simulink model "slrt_induction_2level_inverter"  (R2022b)
settings: Solver=FixedStepAuto  StartTime=0.0  StopTime=0.25  RelTol=1e-3  EnableMultiTasking=on
PreLoadFcn:
  | Ts = 1e-4;
  | Tcpu = 50e-6; %Controller sample time
  | 
  | % PMSM parameters
  | PM = 0.03; % Permanent magnet flux linkage
  | Ld = 2e-4;  % d-axis inductance
  | Lq = 2e-4;  % q-axis inductance
  | L0 = 2e-4;  % 0-axis inductance
  | Rs = 0.013; % Stator resistance
  | N = 6; % Number of pole pairs
  | J = 0.2; % Moment of inertia
  | 
  | % encoder parameters
  | numSlits = 2000; % number of slits
  | pulseSigOffset = 0; % index pulse signal offset
  | shaftInitPos = 0; % motor shaft initial position
  | 
  | % DAC parameters
  | gain = 0.1;
  | bias = 0;
  | 
  | % circuit parameters
  | Vdc = 48;
  | 
  | % real-time parameters
  | ts_FPGA_clk = 5e-9;
  | ts_FPGA_mdl = 1e-6;
  | 
  | % Real-time processor or embedded controller
  | RTorTTL = 1; % 1: Real-time processor,    0: embedded controller
  | 
  | % sample times
  | f_base = 200e6;
  | PWM_frequency = 20e3;
  | ts_FPGA_clk = 1/f_base;
  | ts_FPGA_mdl =1e-6;
undefined symbols (not defined in the file or in its folder): DiscIntNeverNeededParam
libraries: simulink x7, hdlsllib x3, slrtencoderlib x2, slrtresolverlib x2, mcbhdlplantlib x1, slrthdlutillib x1, slrt2levelinverterlib x1
(part 1 of 2)
settings Model: Creator=chrisz  LastModifiedBy=chrisz
settings OptimizationCC: BlockReduction=off  ConditionallyExecuteInputs=off  DefaultParameterBehavior=Inlined
settings DebuggingCC: AlgebraicLoopMsg=error  SingleTaskRateTransMsg=error
settings HardwareCC: ProdBitPerPointer=32  ProdBitPerSizeT=32  ProdBitPerPtrDiffT=32  ProdLargestAtomicFloat=None  ProdIntDivRoundTo=Undefined  ProdEndianess=Unspecified  ProdWordSize=32  ProdHWDeviceType=ASIC/FPGA->ASIC/FPGA  TargetBitPerPointer=64  TargetBitPerSizeT=64  TargetBitPerPtrDiffT=64  TargetLongLongMode=on  TargetIntDivRoundTo=Zero  TargetEndianess=LittleEndian  TargetWordSize=64  TargetHWDeviceType=Custom Processor->MATLAB Host Computer  ProdEqTarget=off
settings ModelReferenceCC: EnableRefExpFcnMdlSchedulingChecks=on

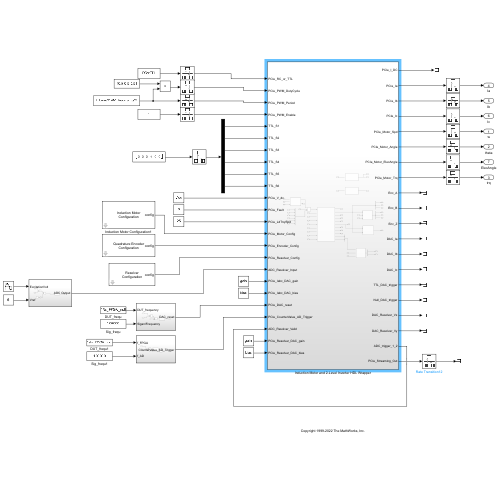
[thumbnail: Simulink's stored preview of the top-level diagram]
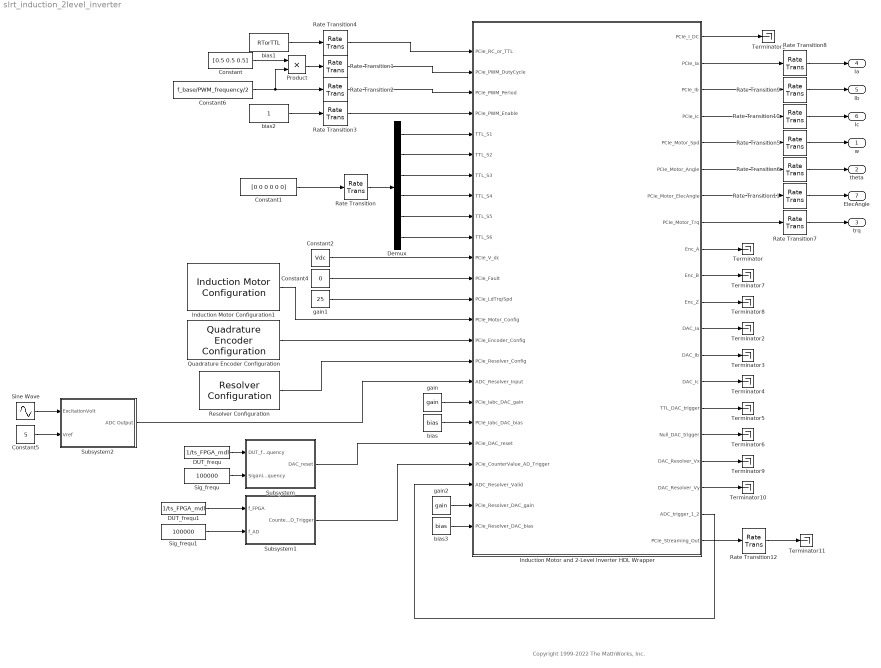
== system slrt_induction_2level_inverter ==
  note: Copyright 1999-2022 The MathWorks, Inc.
  Constant : Constant  Value=[0.5 0.5 0.5]  OutDataTypeStr=single  SampleTime=ts_FPGA_mdl
  Constant1 : Constant  Value=[0 0 0 0 0 0]  OutDataTypeStr=boolean  SampleTime=-1
  Constant2 : Constant  Value=Vdc  OutDataTypeStr=single  SampleTime=ts_FPGA_mdl
  Constant4 : Constant  Value=0  OutDataTypeStr=uint32  SampleTime=ts_FPGA_mdl
  Constant5 : Constant  Value=5  SampleTime=ts_FPGA_mdl
  Constant6 : Constant  Value=f_base/PWM_frequency/2  OutDataTypeStr=uint32  SampleTime=ts_FPGA_mdl
  DUT_frequ : Constant  Value=1/ts_FPGA_mdl  SampleTime=ts_FPGA_mdl
  DUT_frequ1 : Constant  Value=1/ts_FPGA_mdl  SampleTime=ts_FPGA_mdl
  Demux : Demux  Outputs=6
  Induction Motor Configuration1 : mcbhdlplantlib/Induction Motor Configuration  portConfig=Torque  Tw_mode=0  Ts=1e-6  P=2  Rs=1.77  Lls=0.0139  Rr=1.34  Llr=0.0121  Lm=0.3876  J=0.001  B=0  f=0
  Induction Motor and 2-Level Inverter HDL Wrapper : Subsystem
  Product : Product  OutDataTypeStr=uint32
  Quadrature Encoder Configuration : slrtencoderlib/Quadrature Encoder Configuration  NPulses=2000  zOffset=0  Ts=1e-6
  Rate Transition{,1..4} (5 alike) : RateTransition  OutPortSampleTime=ts_FPGA_clk
  Rate Transition{5..12} (8 alike) : RateTransition  OutPortSampleTime=Tcpu
  Resolver Configuration : slrtresolverlib/Resolver Configuration  Ts=1e-6  R=0.5  N=1  ADCrefV=5  ADCbits=12  totalADCCounts=4096
  Sig_frequ : Constant  Value=100000  VectorParams1D=off  SampleTime=ts_FPGA_mdl
  Sig_frequ1 : Constant  Value=100000  VectorParams1D=off  SampleTime=ts_FPGA_mdl
  Sine Wave : Sin  Amplitude=5  Frequency=62830  SampleTime=ts_FPGA_mdl
  Subsystem : Subsystem
  Subsystem1 : Subsystem
  Subsystem2 : Subsystem
  Terminator{,1..11} (12 alike) : Terminator
  bias : Constant  Value=bias  OutDataTypeStr=single  SampleTime=ts_FPGA_mdl
  bias1 : Constant  Value=RTorTTL  OutDataTypeStr=single  SampleTime=ts_FPGA_mdl
  bias2 : Constant  OutDataTypeStr=boolean  SampleTime=ts_FPGA_mdl
  bias3 : Constant  Value=bias  OutDataTypeStr=single  SampleTime=ts_FPGA_mdl
  gain : Constant  Value=gain  OutDataTypeStr=single  SampleTime=ts_FPGA_mdl
  gain1 : Constant  Value=25  OutDataTypeStr=single  SampleTime=ts_FPGA_mdl
  gain2 : Constant  Value=gain  OutDataTypeStr=single  SampleTime=ts_FPGA_mdl
  w : Outport
  theta : Outport  Port=2
  trq : Outport  Port=3
  Ia : Outport  Port=4
  Ib : Outport  Port=5
  Ic : Outport  Port=6
  ElecAngle : Outport  Port=7
  wires:
  bias1/1 -> Rate Transition4/1
  bias2/1 -> Rate Transition3/1
  Constant6/1 -> Product/2, Rate Transition2/1
  Product/1 -> Rate Transition1/1
  Constant/1 -> Product/1
  gain/1 -> Induction Motor and 2-Level Inverter HDL Wrapper/18(PCIe_Iabc_DAC_gain)
  bias/1 -> Induction Motor and 2-Level Inverter HDL Wrapper/19(PCIe_Iabc_DAC_bias)
  Rate Transition4/1 -> Induction Motor and 2-Level Inverter HDL Wrapper/1(PCIe_RC_or_TTL)
  Rate Transition3/1 -> Induction Motor and 2-Level Inverter HDL Wrapper/4(PCIe_PWM_Enable)
  Rate Transition2/1 -> Induction Motor and 2-Level Inverter HDL Wrapper/3(PCIe_PWM_Period)
  Rate Transition1/1 -> Induction Motor and 2-Level Inverter HDL Wrapper/2(PCIe_PWM_DutyCycle)
  Rate Transition/1 -> Demux/1
  Demux/1 -> Induction Motor and 2-Level Inverter HDL Wrapper/5(TTL_S1)
  Demux/2 -> Induction Motor and 2-Level Inverter HDL Wrapper/6(TTL_S2)
  Demux/3 -> Induction Motor and 2-Level Inverter HDL Wrapper/7(TTL_S3)
  Demux/4 -> Induction Motor and 2-Level Inverter HDL Wrapper/8(TTL_S4)
  Demux/5 -> Induction Motor and 2-Level Inverter HDL Wrapper/9(TTL_S5)
  Demux/6 -> Induction Motor and 2-Level Inverter HDL Wrapper/10(TTL_S6)
  Constant1/1 -> Rate Transition/1
  Constant2/1 -> Induction Motor and 2-Level Inverter HDL Wrapper/11(PCIe_V_dc)
  Constant4/1 -> Induction Motor and 2-Level Inverter HDL Wrapper/12(PCIe_Fault)
  gain1/1 -> Induction Motor and 2-Level Inverter HDL Wrapper/13(PCIe_LdTrq/Spd)
  DUT_frequ/1 -> Subsystem/1(DUT_frequency)
  Sig_frequ/1 -> Subsystem/2(SiganlFrequency)
  Subsystem/1(DAC_reset) -> Induction Motor and 2-Level Inverter HDL Wrapper/20(PCIe_DAC_reset)
  Rate Transition6/1 -> theta/1
  Induction Motor and 2-Level Inverter HDL Wrapper/9(Enc_A) -> Terminator/1
  Rate Transition7/1 -> trq/1
  Induction Motor and 2-Level Inverter HDL Wrapper/12(DAC_Ia) -> Terminator2/1
  Induction Motor and 2-Level Inverter HDL Wrapper/1(PCIe_I_DC) -> Terminator1/1
  Induction Motor and 2-Level Inverter HDL Wrapper/10(Enc_B) -> Terminator7/1
  Induction Motor and 2-Level Inverter HDL Wrapper/14(DAC_Ic) -> Terminator4/1
  Rate Transition5/1 -> w/1
  Rate Transition10/1 -> Ic/1
  Induction Motor and 2-Level Inverter HDL Wrapper/15(TTL_DAC_trigger) -> Terminator5/1
  Induction Motor and 2-Level Inverter HDL Wrapper/13(DAC_Ib) -> Terminator3/1
  Induction Motor and 2-Level Inverter HDL Wrapper/16(Null_DAC_trigger) -> Terminator6/1
  Rate Transition9/1 -> Ib/1
  Rate Transition8/1 -> Ia/1
  Induction Motor and 2-Level Inverter HDL Wrapper/5(PCIe_Motor_Spd) -> Rate Transition5/1
  Induction Motor and 2-Level Inverter HDL Wrapper/6(PCIe_Motor_Angle) -> Rate Transition6/1
  Induction Motor and 2-Level Inverter HDL Wrapper/8(PCIe_Motor_Trq) -> Rate Transition7/1
  Induction Motor and 2-Level Inverter HDL Wrapper/2(PCIe_Ia) -> Rate Transition8/1
  Induction Motor and 2-Level Inverter HDL Wrapper/3(PCIe_Ib) -> Rate Transition9/1
  Induction Motor and 2-Level Inverter HDL Wrapper/4(PCIe_Ic) -> Rate Transition10/1
  Induction Motor and 2-Level Inverter HDL Wrapper/11(Enc_Z) -> Terminator8/1
  Induction Motor and 2-Level Inverter HDL Wrapper/17(DAC_Resolver_Vx) -> Terminator9/1
  Induction Motor and 2-Level Inverter HDL Wrapper/18(DAC_Resolver_Vy) -> Terminator10/1
  Quadrature Encoder Configuration/1 -> Induction Motor and 2-Level Inverter HDL Wrapper/15(PCIe_Encoder_Config)
  Induction Motor Configuration1/1 -> Induction Motor and 2-Level Inverter HDL Wrapper/14(PCIe_Motor_Config)
  Resolver Configuration/1 -> Induction Motor and 2-Level Inverter HDL Wrapper/16(PCIe_Resolver_Config)
  Subsystem1/1(CounterValue_AD_Trigger) -> Induction Motor and 2-Level Inverter HDL Wrapper/21(PCIe_CounterValue_AD_Trigger)
  Induction Motor and 2-Level Inverter HDL Wrapper/19(ADC_trigger_1_2) -> Induction Motor and 2-Level Inverter HDL Wrapper/22(ADC_Resolver_Valid)
  Sig_frequ1/1 -> Subsystem1/2(f_AD)
  DUT_frequ1/1 -> Subsystem1/1(f_FPGA)
  Sine Wave/1 -> Subsystem2/1(ExcitationVolt)
  Constant5/1 -> Subsystem2/2(Vref)
  Subsystem2/1(ADC Output) -> Induction Motor and 2-Level Inverter HDL Wrapper/17(ADC_Resolver_Input)
  Rate Transition11/1 -> ElecAngle/1
  Induction Motor and 2-Level Inverter HDL Wrapper/7(PCIe_Motor_ElecAngle) -> Rate Transition11/1
  gain2/1 -> Induction Motor and 2-Level Inverter HDL Wrapper/23(PCIe_Resolver_DAC_gain)
  bias3/1 -> Induction Motor and 2-Level Inverter HDL Wrapper/24(PCIe_Resolver_DAC_bias)
  Induction Motor and 2-Level Inverter HDL Wrapper/20(PCIe_Streaming_Out) -> Rate Transition12/1
  Rate Transition12/1 -> Terminator11/1

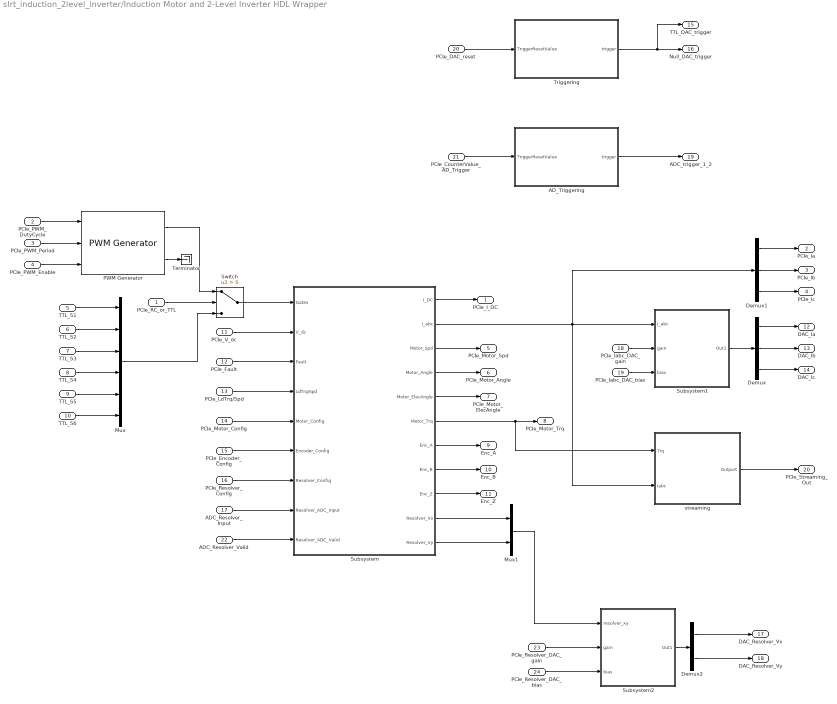
== system slrt_induction_2level_inverter/Induction Motor and 2-Level Inverter HDL Wrapper ==
  PCIe_RC_or_TTL : Inport
  PCIe_PWM_DutyCycle : Inport  Port=2
  PCIe_PWM_Period : Inport  Port=3
  PCIe_PWM_Enable : Inport  Port=4
  TTL_S1 : Inport  Port=5
  TTL_S2 : Inport  Port=6
  TTL_S3 : Inport  Port=7
  TTL_S4 : Inport  Port=8
  TTL_S5 : Inport  Port=9
  TTL_S6 : Inport  Port=10
  PCIe_V_dc : Inport  Port=11
  PCIe_Fault : Inport  Port=12
  PCIe_LdTrq/Spd : Inport  Port=13
  PCIe_Motor_Config : Inport  Port=14
  PCIe_Encoder_Config : Inport  Port=15
  PCIe_Resolver_Config : Inport  Port=16
  ADC_Resolver_Input : Inport  Port=17
  PCIe_Iabc_DAC_gain : Inport  Port=18
  PCIe_Iabc_DAC_bias : Inport  Port=19
  PCIe_DAC_reset : Inport  Port=20
  PCIe_CounterValue_AD_Trigger : Inport  Port=21  OutDataTypeStr=uint32
  ADC_Resolver_Valid : Inport  Port=22
  PCIe_Resolver_DAC_gain : Inport  Port=23
  PCIe_Resolver_DAC_bias : Inport  Port=24
  AD_Triggering : Subsystem
  Demux : Demux  Outputs=3
  Demux1 : Demux  Outputs=3
  Demux2 : Demux  Outputs=2
  Mux : Mux  Inputs=6
  Mux1 : Mux  Inputs=2
  PWM Generator : slrthdlutillib/PWM Generator
  Subsystem : Subsystem
  Subsystem1 : Subsystem
  Subsystem2 : Subsystem
  Switch : Switch  Criteria=u2 > Threshold  SaturateOnIntegerOverflow=off  InputSameDT=off
  Terminator : Terminator
  Triggering : Subsystem
  streaming : Subsystem
  PCIe_I_DC : Outport
  PCIe_Ia : Outport  Port=2
  PCIe_Ib : Outport  Port=3
  PCIe_Ic : Outport  Port=4
  PCIe_Motor_Spd : Outport  Port=5
  PCIe_Motor_Angle : Outport  Port=6
  PCIe_Motor_ElecAngle : Outport  Port=7
  PCIe_Motor_Trq : Outport  Port=8
  Enc_A : Outport  Port=9
  Enc_B : Outport  Port=10
  Enc_Z : Outport  Port=11
  DAC_Ia : Outport  Port=12
  DAC_Ib : Outport  Port=13
  DAC_Ic : Outport  Port=14
  TTL_DAC_trigger : Outport  Port=15
  Null_DAC_trigger : Outport  Port=16
  DAC_Resolver_Vx : Outport  Port=17
  DAC_Resolver_Vy : Outport  Port=18
  ADC_trigger_1_2 : Outport  Port=19  OutDataTypeStr=boolean
  PCIe_Streaming_Out : Outport  Port=20
  wires:
  Subsystem/7(Enc_A) -> Enc_A/1
  TTL_S2/1 -> Mux/2
  Demux1/1 -> PCIe_Ia/1
  PCIe_PWM_DutyCycle/1 -> PWM Generator/1
  TTL_S5/1 -> Mux/5
  Subsystem/2(I_abc) -> Demux1/1, streaming/2(Iabc), Subsystem1/1(I_abc)
  Subsystem/6(Motor_Trq) -> streaming/1(Trq), PCIe_Motor_Trq/1
  Subsystem/4(Motor_Angle) -> PCIe_Motor_Angle/1
  Subsystem/1(I_DC) -> PCIe_I_DC/1
  PCIe_Encoder_Config/1 -> Subsystem/6(Encoder_Config)
  PCIe_Iabc_DAC_bias/1 -> Subsystem1/3(bias)
  Subsystem/3(Motor_Spd) -> PCIe_Motor_Spd/1
  Subsystem/8(Enc_B) -> Enc_B/1
  PCIe_V_dc/1 -> Subsystem/2(V_dc)
  PWM Generator/1 -> Switch/1
  Triggering/1(trigger) -> Null_DAC_trigger/1, TTL_DAC_trigger/1
  TTL_S6/1 -> Mux/6
  Subsystem/9(Enc_Z) -> Enc_Z/1
  PCIe_LdTrq/Spd/1 -> Subsystem/4(LdTrq/Spd)
  TTL_S1/1 -> Mux/1
  Demux1/3 -> PCIe_Ic/1
  Demux1/2 -> PCIe_Ib/1
  PCIe_RC_or_TTL/1 -> Switch/2
  PCIe_Motor_Config/1 -> Subsystem/5(Motor_Config)
  Demux/1 -> DAC_Ia/1
  Mux/1 -> Switch/3
  PCIe_PWM_Period/1 -> PWM Generator/2
  TTL_S4/1 -> Mux/4
  PCIe_Fault/1 -> Subsystem/3(Fault)
  PCIe_DAC_reset/1 -> Triggering/1(TriggerResetValue)
  PCIe_Iabc_DAC_gain/1 -> Subsystem1/2(gain)
  PCIe_PWM_Enable/1 -> PWM Generator/3
  Demux/2 -> DAC_Ib/1
  Switch/1 -> Subsystem/1(Gates)
  Subsystem1/1(Out1) -> Demux/1
  TTL_S3/1 -> Mux/3
  Demux/3 -> DAC_Ic/1
  PCIe_Resolver_Config/1 -> Subsystem/7(Resolver_Config)
  ADC_Resolver_Input/1 -> Subsystem/8(Resolver_ADC_Input)
  PCIe_CounterValue_AD_Trigger/1 -> AD_Triggering/1(TriggerResetValue)
  AD_Triggering/1(trigger) -> ADC_trigger_1_2/1
  ADC_Resolver_Valid/1 -> Subsystem/9(Resolver_ADC_Valid)
  Subsystem/5(Motor_ElecAngle) -> PCIe_Motor_ElecAngle/1
  streaming/1(Outport) -> PCIe_Streaming_Out/1
  Subsystem/10(Resolver_Vx) -> Mux1/1
  Subsystem/11(Resolver_Vy) -> Mux1/2
  Mux1/1 -> Subsystem2/1(resolver_xy)
  PCIe_Resolver_DAC_gain/1 -> Subsystem2/2(gain)
  PCIe_Resolver_DAC_bias/1 -> Subsystem2/3(bias)
  Subsystem2/1(Out1) -> Demux2/1
  Demux2/1 -> DAC_Resolver_Vx/1
  Demux2/2 -> DAC_Resolver_Vy/1
  PWM Generator/2 -> Terminator/1

== system slrt_induction_2level_inverter/Subsystem ==
  DUT_frequency : Inport
  SiganlFrequency : Inport  Port=2
  Add : Sum  Inputs=+-
  Data Type Conversion : DataTypeConversion  OutDataTypeStr=uint16  SaturateOnIntegerOverflow=off  RndMeth=Floor
  Divide : Product  Inputs=*/
  constant : Constant  VectorParams1D=off  SampleTime=-1
  DAC_reset : Outport
  wires:
  DUT_frequency/1 -> Divide/1
  constant/1 -> Add/2
  Data Type Conversion/1 -> DAC_reset/1
  Divide/1 -> Add/1
  Add/1 -> Data Type Conversion/1
  SiganlFrequency/1 -> Divide/2

== system slrt_induction_2level_inverter/Subsystem1 ==
  f_FPGA : Inport
  f_AD : Inport  Port=2
  Add : Sum  Inputs=+-  AccumDataTypeStr=uint32
  Data Type Conversion : DataTypeConversion  OutDataTypeStr=uint32  SaturateOnIntegerOverflow=off  RndMeth=Floor
  Divide : Product  Inputs=*/
  constant : Constant  VectorParams1D=off  OutDataTypeStr=uint32  SampleTime=-1
  CounterValue_AD_Trigger : Outport
  wires:
  f_AD/1 -> Divide/2
  f_FPGA/1 -> Divide/1
  Divide/1 -> Data Type Conversion/1
  Data Type Conversion/1 -> Add/1
  constant/1 -> Add/2
  Add/1 -> CounterValue_AD_Trigger/1

== system slrt_induction_2level_inverter/Subsystem2 ==
  ExcitationVolt : Inport
  Vref : Inport  Port=2
  Constant : Constant  Value=2^16  SampleTime=-1
  Data Type Conversion : DataTypeConversion  OutDataTypeStr=int16  RndMeth=Nearest
  Divide : Product  Inputs=*/
  Gain : Gain  Gain=0.5
  Product : Product
  ADC Output : Outport
  wires:
  ExcitationVolt/1 -> Divide/1
  Vref/1 -> Divide/2
  Constant/1 -> Gain/1
  Divide/1 -> Product/1
  Gain/1 -> Product/2
  Product/1 -> Data Type Conversion/1
  Data Type Conversion/1 -> ADC Output/1

== system slrt_induction_2level_inverter/Induction Motor and 2-Level Inverter HDL Wrapper/AD_Triggering ==
  TriggerResetValue : Inport
  HDL Counter : hdlsllib/Sources/HDL Counter  CountType=Free running  CountInit=0  CountStep=1  CountMax=25  CountFromType=Initial value  CountFrom=0  CountResetPort=on  CountLoadPort=off  CountEnbPort=off  CountDirPort=off  CountHitOutputPort=off  CountDataType=Unsigned  CountWordLen=32  CountFracLen=0  CountSampTime=1
  Relational Operator : RelationalOperator  Operator=<=  OutDataTypeStr=boolean  InputSameDT=off
  Unit Delay : UnitDelay  SampleTime=-1  HasFrameUpgradeWarning=on
  trigger : Outport
  wires:
  TriggerResetValue/1 -> Relational Operator/1
  HDL Counter/1 -> Relational Operator/2
  Relational Operator/1 -> HDL Counter/1, Unit Delay/1
  Unit Delay/1 -> trigger/1

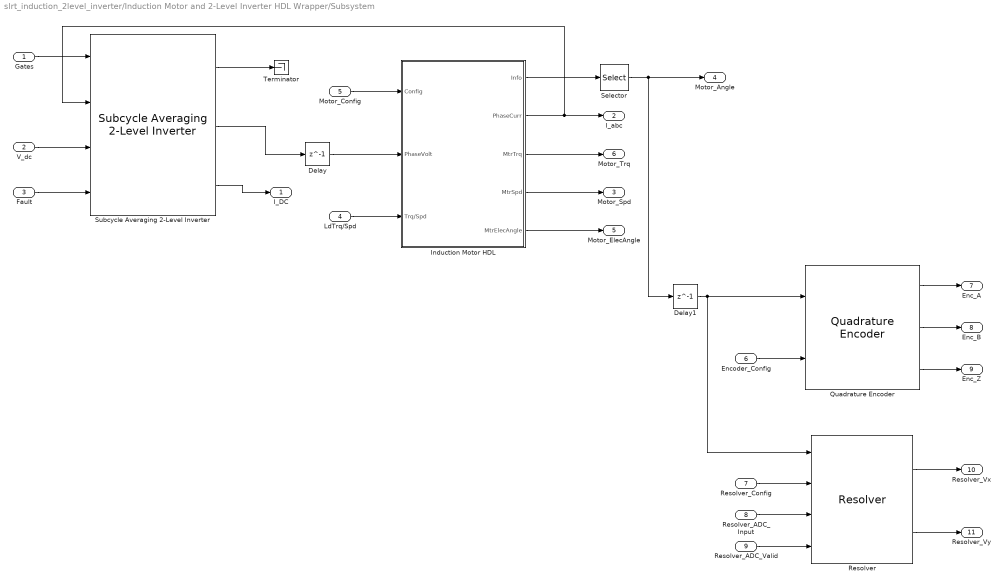
== system slrt_induction_2level_inverter/Induction Motor and 2-Level Inverter HDL Wrapper/Subsystem ==
  Gates : Inport
  V_dc : Inport  Port=2
  Fault : Inport  Port=3
  LdTrq/Spd : Inport  Port=4
  Motor_Config : Inport  Port=5
  Encoder_Config : Inport  Port=6
  Resolver_Config : Inport  Port=7
  Resolver_ADC_Input : Inport  Port=8
  Resolver_ADC_Valid : Inport  Port=9
  Delay : Delay  DelayLength=1
  Delay1 : Delay  DelayLength=1
  Induction Motor HDL : Subsystem  mask{Ts=1e-6}
      mask prompts: Ts "mcb:PlantLib:IMHDLPrm"
      mask DialogControl DescGroupVar Prompt: mcb:PlantLib:IMHDLTitle
      mask DialogControl DescTextVar Prompt: mcb:PlantLib:IMHDLDes
      mask DialogControl Ts Prompt: Sample time (s):
      mask Display:
      | disp('Induction\nMotor HDL');
      | port_label('input',1,'Config');
      | port_label('input',2,'PhaseVolt');
      | port_label('input',3,'LdTrq/Spd');
      | port_label('output',1,'Info');
      | port_label('output',2,'PhaseCurr');
      | port_label('output',3,'Torque');
      | port_label('output',4,'Speed');
      | port_label('output',5,'MtrElecAngle');
  Quadrature Encoder : slrtencoderlib/Quadrature Encoder
  Resolver : slrtresolverlib/Resolver  Ts=1e-6
  Selector : Selector  InputPortWidth=19  IndexOptions=Index vector (dialog)  Indices=[9]  OutputSizes=1
  Subcycle Averaging 2-Level Inverter : slrt2levelinverterlib/Subcycle Averaging 2-Level Inverter   rSwitch=0.001  vfSwitch=0.1  rDiode=0.001  vfDiode=0.8  rSnub=100  ts_Model=ts_FPGA_mdl  ts_FPGA=ts_FPGA_clk
  Terminator : Terminator
  I_DC : Outport
  I_abc : Outport  Port=2
  Motor_Spd : Outport  Port=3
  Motor_Angle : Outport  Port=4
  Motor_ElecAngle : Outport  Port=5
  Motor_Trq : Outport  Port=6
  Enc_A : Outport  Port=7
  Enc_B : Outport  Port=8
  Enc_Z : Outport  Port=9
  Resolver_Vx : Outport  Port=10
  Resolver_Vy : Outport  Port=11
  wires:
  Motor_Config/1 -> Induction Motor HDL/1(Config)
  Subcycle Averaging 2-Level Inverter/3 -> I_DC/1
  V_dc/1 -> Subcycle Averaging 2-Level Inverter/3
  Induction Motor HDL/2(PhaseCurr) -> Subcycle Averaging 2-Level Inverter/2, I_abc/1
  Quadrature Encoder/2 -> Enc_B/1
  Fault/1 -> Subcycle Averaging 2-Level Inverter/4
  Quadrature Encoder/1 -> Enc_A/1
  Induction Motor HDL/3(MtrTrq) -> Motor_Trq/1
  LdTrq/Spd/1 -> Induction Motor HDL/3(Trq/Spd)
  Quadrature Encoder/3 -> Enc_Z/1
  Induction Motor HDL/4(MtrSpd) -> Motor_Spd/1
  Encoder_Config/1 -> Quadrature Encoder/2
  Gates/1 -> Subcycle Averaging 2-Level Inverter/1
  Resolver_Config/1 -> Resolver/2
  Resolver_ADC_Input/1 -> Resolver/3
  Resolver/1 -> Resolver_Vx/1
  Resolver/2 -> Resolver_Vy/1
  Resolver_ADC_Valid/1 -> Resolver/4
  Subcycle Averaging 2-Level Inverter/1 -> Terminator/1
  Induction Motor HDL/1(Info) -> Selector/1
  Induction Motor HDL/5(MtrElecAngle) -> Motor_ElecAngle/1
  Subcycle Averaging 2-Level Inverter/2 -> Delay/1
  Delay/1 -> Induction Motor HDL/2(PhaseVolt)
  Selector/1 -> Delay1/1, Motor_Angle/1
  Delay1/1 -> Resolver/1, Quadrature Encoder/1

== system slrt_induction_2level_inverter/Induction Motor and 2-Level Inverter HDL Wrapper/Subsystem1 ==
  I_abc : Inport
  gain : Inport  Port=2
  bias : Inport  Port=3
  Add : Sum
  Data Type Conversion : DataTypeConversion  OutDataTypeStr=int16  SaturateOnIntegerOverflow=off  RndMeth=Floor
  Gain : Gain  Gain=2^15/10
  Product : Product
  Unit Delay : UnitDelay  SampleTime=-1  HasFrameUpgradeWarning=on
  Out1 : Outport
  wires:
  I_abc/1 -> Unit Delay/1
  Unit Delay/1 -> Product/1
  gain/1 -> Product/2
  Product/1 -> Add/1
  bias/1 -> Add/2
  Add/1 -> Gain/1
  Gain/1 -> Data Type Conversion/1
  Data Type Conversion/1 -> Out1/1

== system slrt_induction_2level_inverter/Induction Motor and 2-Level Inverter HDL Wrapper/Subsystem2 ==
  resolver_xy : Inport
  gain : Inport  Port=2
  bias : Inport  Port=3
  Add : Sum
  Data Type Conversion : DataTypeConversion  OutDataTypeStr=int16  SaturateOnIntegerOverflow=off  RndMeth=Floor
  Gain : Gain  Gain=2^15/10
  Product : Product
  Unit Delay : UnitDelay  SampleTime=-1  HasFrameUpgradeWarning=on
  Out1 : Outport
  wires:
  resolver_xy/1 -> Unit Delay/1
  Unit Delay/1 -> Product/1
  gain/1 -> Product/2
  Product/1 -> Add/1
  bias/1 -> Add/2
  Add/1 -> Gain/1
  Gain/1 -> Data Type Conversion/1
  Data Type Conversion/1 -> Out1/1

== system slrt_induction_2level_inverter/Induction Motor and 2-Level Inverter HDL Wrapper/Triggering ==
  TriggerResetValue : Inport
  HDL Counter : hdlsllib/Sources/HDL Counter  CountType=Free running  CountInit=0  CountStep=1  CountMax=25  CountFromType=Initial value  CountFrom=0  CountResetPort=on  CountLoadPort=off  CountEnbPort=off  CountDirPort=off  CountHitOutputPort=off  CountDataType=Unsigned  CountWordLen=16  CountFracLen=0  CountSampTime=1
  Relational Operator : RelationalOperator  Operator===  OutDataTypeStr=boolean  InputSameDT=off
  Unit Delay : UnitDelay  SampleTime=-1  HasFrameUpgradeWarning=on
  trigger : Outport
  wires:
  TriggerResetValue/1 -> Relational Operator/1
  HDL Counter/1 -> Relational Operator/2
  Relational Operator/1 -> HDL Counter/1, Unit Delay/1
  Unit Delay/1 -> trigger/1

== system slrt_induction_2level_inverter/Induction Motor and 2-Level Inverter HDL Wrapper/streaming ==
  Trq : Inport
  Iabc : Inport  Port=2
  Compare To Zero : simulink/Logic and Bit Operations/Compare To Zero  relop===  OutDataTypeStr=boolean
  Counter Limited : simulink/Sources/Counter Limited  uplimit=49  tsamp=ts_FPGA_mdl
  Mux : Mux  Inputs=3
  Rate Transition : RateTransition
  Rate Transition3 : RateTransition
  Rate Transition4 : RateTransition
  Selector : Selector  InputPortWidth=3  IndexOptions=Index vector (dialog)  Indices=[1]  OutputSizes=1
  Selector1 : Selector  InputPortWidth=3  IndexOptions=Index vector (dialog)  Indices=[2]  OutputSizes=1
  Tapped Delay : simulink/Discrete/Tapped Delay  vinit=0.0  samptime=ts_FPGA_mdl  NumDelays=50  DelayOrder=Oldest  includeCurrent=off
  Tapped Delay3 : simulink/Discrete/Tapped Delay  vinit=0.0  samptime=ts_FPGA_mdl  NumDelays=50  DelayOrder=Oldest  includeCurrent=off
  Tapped Delay4 : simulink/Discrete/Tapped Delay  vinit=0.0  samptime=ts_FPGA_mdl  NumDelays=50  DelayOrder=Oldest  includeCurrent=off
  Unit Delay Enabled Synchronous : hdlsllib/Discrete/Unit Delay Enabled Synchronous  InitialCondition=0.0  SampleTime=-1
  Outport : Outport
  wires:
  Iabc/1 -> Rate Transition4/1, Rate Transition/1
  Trq/1 -> Rate Transition3/1
  Rate Transition3/1 -> Tapped Delay/1
  Rate Transition/1 -> Selector/1
  Rate Transition4/1 -> Selector1/1
  Selector/1 -> Tapped Delay3/1
  Selector1/1 -> Tapped Delay4/1
  Tapped Delay/1 -> Mux/1
  Tapped Delay3/1 -> Mux/2
  Tapped Delay4/1 -> Mux/3
  Mux/1 -> Unit Delay Enabled Synchronous/1
  Counter Limited/1 -> Compare To Zero/1
  Compare To Zero/1 -> Unit Delay Enabled Synchronous/2
  Unit Delay Enabled Synchronous/1 -> Outport/1

== system slrt_induction_2level_inverter/Induction Motor and 2-Level Inverter HDL Wrapper/Subsystem/Induction Motor HDL ==
  Config : Inport  Unit=V  SampleTime=Ts
  PhaseVolt : Inport  Port=2  Unit=V  SampleTime=Ts
  Trq/Spd : Inport  Port=3  Unit=N*m  SampleTime=Ts
  IM HDL : Subsystem  VariantControl=imVariant==imEnum.VelocityInput
  Info : Outport  SampleTime=Ts  VectorParamsAs1DForOutWhenUnconnected=off
  PhaseCurr : Outport  Port=2  Unit=A  SampleTime=Ts  VectorParamsAs1DForOutWhenUnconnected=off
  MtrTrq : Outport  Port=3  Unit=rad/s  SampleTime=Ts  VectorParamsAs1DForOutWhenUnconnected=off
  MtrSpd : Outport  Port=4  Unit=rad/s  SampleTime=Ts  VectorParamsAs1DForOutWhenUnconnected=off
  MtrElecAngle : Outport  Port=5  Unit=rad/s  SampleTime=Ts  VectorParamsAs1DForOutWhenUnconnected=off
  wires:
  IM HDL/5(MtrElecAngle) -> MtrElecAngle/1
  IM HDL/3(MtrTrq) -> MtrTrq/1
  Config/1 -> IM HDL/1(Config)
  IM HDL/1(Info) -> Info/1
  Trq/Spd/1 -> IM HDL/3(Trq/Spd)
  PhaseVolt/1 -> IM HDL/2(PhaseVolt)
  IM HDL/2(PhaseCurr) -> PhaseCurr/1
  IM HDL/4(MtrSpd) -> MtrSpd/1

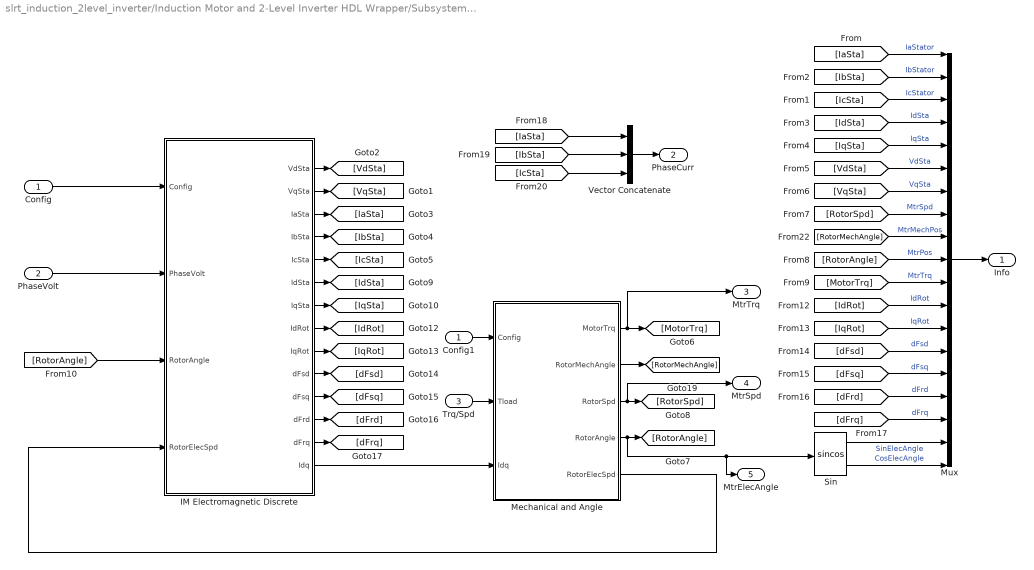
== system slrt_induction_2level_inverter/Induction Motor and 2-Level Inverter HDL Wrapper/Subsystem/Induction Motor HDL/IM HDL ==
  Config : Inport
  PhaseVolt : Inport  Port=2
  Trq/Spd : Inport  Port=3
  Config1 : InportShadow
  IM Electromagnetic Discrete : Subsystem
  Mechanical and Angle : Subsystem
  Mux : Mux  Inputs=19
  Sin : Trigonometry  Operator=sincos
  Vector Concatenate : Concatenate  NumInputs=3
  Info : Outport  VectorParamsAs1DForOutWhenUnconnected=off
  PhaseCurr : Outport  Port=2  VectorParamsAs1DForOutWhenUnconnected=off
  MtrTrq : Outport  Port=3  VectorParamsAs1DForOutWhenUnconnected=off
  MtrSpd : Outport  Port=4  VectorParamsAs1DForOutWhenUnconnected=off
  MtrElecAngle : Outport  Port=5  VectorParamsAs1DForOutWhenUnconnected=off
  wires:
  Sin/2 -> Mux/19  "CosElecAngle"
  Sin/1 -> Mux/18  "SinElecAngle"
  Mechanical and Angle/1(MotorTrq) -> MtrTrq/1, [MotorTrq]
  Mux/1 -> Info/1
  Config1/1 -> Mechanical and Angle/1(Config)
  Config/1 -> IM Electromagnetic Discrete/1(Config)
  IM Electromagnetic Discrete/14(Idq) -> Mechanical and Angle/3(Idq)
  [RotorMechAngle] -> Mux/9  "MtrMechPos"
  Mechanical and Angle/2(RotorMechAngle) -> [RotorMechAngle]
  [MotorTrq] -> Mux/11  "MtrTrq"
  [RotorAngle] -> Mux/10  "MtrPos"
  [RotorSpd] -> Mux/8  "MtrSpd"
  [VqSta] -> Mux/7  "VqSta"
  [VdSta] -> Mux/6  "VdSta"
  [IqSta] -> Mux/5  "IqSta"
  [IdSta] -> Mux/4  "IdSta"
  [IcSta] -> Mux/3  "IcStator"
  [IbSta] -> Mux/2  "IbStator"
  [IaSta] -> Mux/1  "IaStator"
  Trq/Spd/1 -> Mechanical and Angle/2(Tload)
  Mechanical and Angle/4(RotorAngle) -> [RotorAngle], MtrElecAngle/1, Sin/1
  Mechanical and Angle/5(RotorElecSpd) -> IM Electromagnetic Discrete/4(RotorElecSpd)
  Mechanical and Angle/3(RotorSpd) -> MtrSpd/1, [RotorSpd]
  PhaseVolt/1 -> IM Electromagnetic Discrete/2(PhaseVolt)
  [RotorAngle] -> IM Electromagnetic Discrete/3(RotorAngle)
  IM Electromagnetic Discrete/1(VdSta) -> [VdSta]
  IM Electromagnetic Discrete/2(VqSta) -> [VqSta]
  IM Electromagnetic Discrete/3(IaSta) -> [IaSta]
  IM Electromagnetic Discrete/4(IbSta) -> [IbSta]
  IM Electromagnetic Discrete/5(IcSta) -> [IcSta]
  IM Electromagnetic Discrete/6(IdSta) -> [IdSta]
  IM Electromagnetic Discrete/7(IqSta) -> [IqSta]
  IM Electromagnetic Discrete/8(IdRot) -> [IdRot]
  IM Electromagnetic Discrete/9(IqRot) -> [IqRot]
  IM Electromagnetic Discrete/10(dFsd) -> [dFsd]
  IM Electromagnetic Discrete/11(dFsq) -> [dFsq]
  IM Electromagnetic Discrete/12(dFrd) -> [dFrd]
  IM Electromagnetic Discrete/13(dFrq) -> [dFrq]
  [IdRot] -> Mux/12  "IdRot"
  [IqRot] -> Mux/13  "IqRot"
  [dFsd] -> Mux/14  "dFsd"
  [dFsq] -> Mux/15  "dFsq"
  [dFrd] -> Mux/16  "dFrd"
  [dFrq] -> Mux/17  "dFrq"
  Vector Concatenate/1 -> PhaseCurr/1
  [IaSta] -> Vector Concatenate/1
  [IbSta] -> Vector Concatenate/2
  [IcSta] -> Vector Concatenate/3

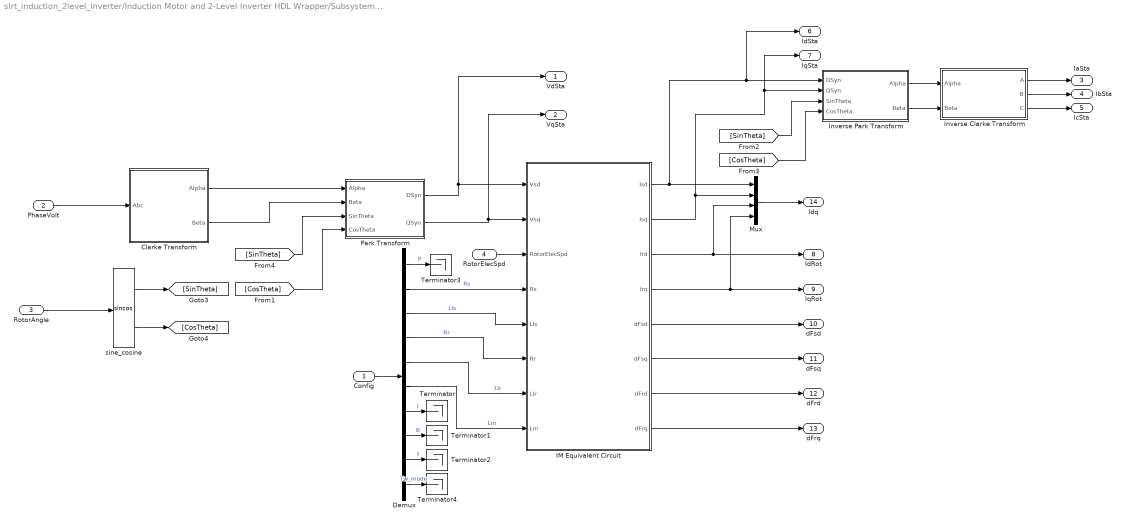
== system slrt_induction_2level_inverter/Induction Motor and 2-Level Inverter HDL Wrapper/Subsystem/Induction Motor HDL/IM HDL/IM Electromagnetic Discrete ==
  Config : Inport
  PhaseVolt : Inport  Port=2
  RotorAngle : Inport  Port=3
  RotorElecSpd : Inport  Port=4
  Clarke Transform : Subsystem
  Demux : Demux  Outputs=10
  IM Equivalent Circuit : Subsystem
  Inverse Clarke Transform : Subsystem
  Inverse Park Transform : Subsystem
  Mux : Mux
  Park Transform : Subsystem
  Terminator{,1..4} (5 alike) : Terminator
  sine_cosine : Trigonometry  Operator=sincos
  VdSta : Outport  VectorParamsAs1DForOutWhenUnconnected=off
  VqSta : Outport  Port=2  VectorParamsAs1DForOutWhenUnconnected=off
  IaSta : Outport  Port=3  VectorParamsAs1DForOutWhenUnconnected=off
  IbSta : Outport  Port=4  VectorParamsAs1DForOutWhenUnconnected=off
  IcSta : Outport  Port=5  VectorParamsAs1DForOutWhenUnconnected=off
  IdSta : Outport  Port=6  VectorParamsAs1DForOutWhenUnconnected=off
  IqSta : Outport  Port=7  VectorParamsAs1DForOutWhenUnconnected=off
  IdRot : Outport  Port=8  VectorParamsAs1DForOutWhenUnconnected=off
  IqRot : Outport  Port=9  VectorParamsAs1DForOutWhenUnconnected=off
  dFsd : Outport  Port=10  VectorParamsAs1DForOutWhenUnconnected=off
  dFsq : Outport  Port=11  VectorParamsAs1DForOutWhenUnconnected=off
  dFrd : Outport  Port=12  VectorParamsAs1DForOutWhenUnconnected=off
  dFrq : Outport  Port=13  VectorParamsAs1DForOutWhenUnconnected=off
  Idq : Outport  Port=14  VectorParamsAs1DForOutWhenUnconnected=off
  wires:
  Demux/3 -> IM Equivalent Circuit/5(Lls)  "Lls"
  Demux/4 -> IM Equivalent Circuit/6(Rr)  "Rr"
  Demux/10 -> Terminator4/1  "Tw_mode"
  Mux/1 -> Idq/1
  Demux/2 -> IM Equivalent Circuit/4(Rs)  "Rs"
  Demux/1 -> Terminator3/1  "P"
  Demux/5 -> IM Equivalent Circuit/7(Llr)  "Llr"
  Demux/7 -> Terminator/1  "J"
  Config/1 -> Demux/1
  Demux/9 -> Terminator2/1  "f"
  Demux/8 -> Terminator1/1  "B"
  Demux/6 -> IM Equivalent Circuit/8(Lm)  "Lm"
  Inverse Park Transform/2(Beta) -> Inverse Clarke Transform/2(Beta)
  Inverse Park Transform/1(Alpha) -> Inverse Clarke Transform/1(Alpha)
  IM Equivalent Circuit/8(dFrq) -> dFrq/1
  IM Equivalent Circuit/7(dFrd) -> dFrd/1
  IM Equivalent Circuit/6(dFsq) -> dFsq/1
  IM Equivalent Circuit/5(dFsd) -> dFsd/1
  Inverse Clarke Transform/1(A) -> IaSta/1
  Inverse Clarke Transform/2(B) -> IbSta/1
  Inverse Clarke Transform/3(C) -> IcSta/1
  RotorAngle/1 -> sine_cosine/1
  RotorElecSpd/1 -> IM Equivalent Circuit/3(RotorElecSpd)
  [SinTheta] -> Inverse Park Transform/3(SinTheta)
  [CosTheta] -> Inverse Park Transform/4(CosTheta)
  sine_cosine/2 -> [CosTheta]
  sine_cosine/1 -> [SinTheta]
  Park Transform/2(QSyn) -> IM Equivalent Circuit/2(Vsq), VqSta/1
  Park Transform/1(DSyn) -> IM Equivalent Circuit/1(Vsd), VdSta/1
  PhaseVolt/1 -> Clarke Transform/1(Abc)
  Clarke Transform/2(Beta) -> Park Transform/2(Beta)
  Clarke Transform/1(Alpha) -> Park Transform/1(Alpha)
  [SinTheta] -> Park Transform/3(SinTheta)
  [CosTheta] -> Park Transform/4(CosTheta)
  IM Equivalent Circuit/1(Isd) -> Inverse Park Transform/1(DSyn), IdSta/1, Mux/1
  IM Equivalent Circuit/4(Irq) -> Mux/4, IqRot/1
  IM Equivalent Circuit/3(Ird) -> Mux/3, IdRot/1
  IM Equivalent Circuit/2(Isq) -> IqSta/1, Inverse Park Transform/2(QSyn), Mux/2

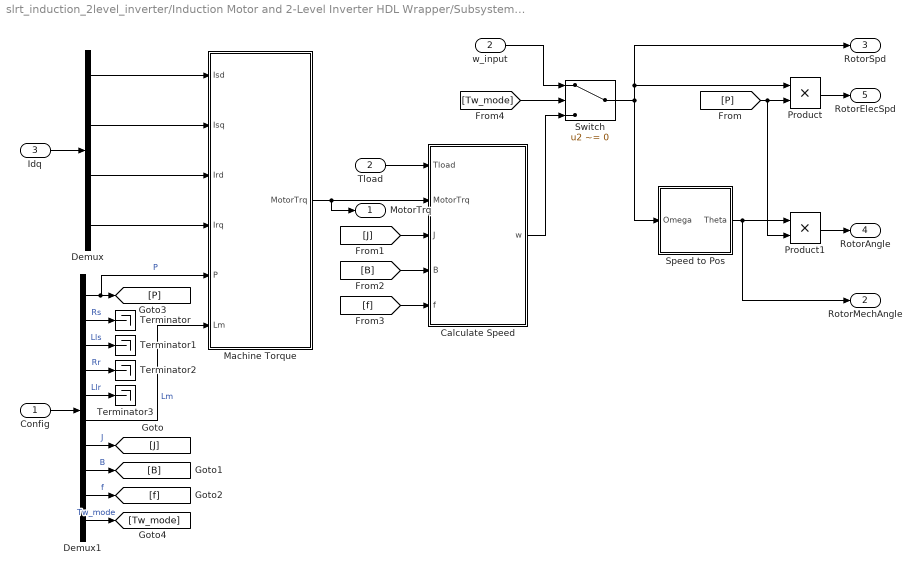
== system slrt_induction_2level_inverter/Induction Motor and 2-Level Inverter HDL Wrapper/Subsystem/Induction Motor HDL/IM HDL/Mechanical and Angle ==
  Config : Inport
  Tload : Inport  Port=2
  Idq : Inport  Port=3
  Calculate Speed : Subsystem
  Demux : Demux
  Demux1 : Demux  Outputs=10
  Machine Torque : Subsystem
  Product : Product  OutDataTypeStr=Inherit: Same as first input
  Product1 : Product  OutDataTypeStr=Inherit: Same as first input
  Speed to Pos : Subsystem  mask{Ts=Ts, U=pi, L=-pi}
      mask prompts: Ts "Sample Time:"; U "Upper Limit:"; L "Lower Limit:"
      mask help: Discrete integrator with wrap
  Switch : Switch  Criteria=u2 ~= 0  SaturateOnIntegerOverflow=off  InputSameDT=off
  Terminator{,1..3} (4 alike) : Terminator
  w_input : InportShadow  Port=2
  MotorTrq : Outport  VectorParamsAs1DForOutWhenUnconnected=off
  RotorMechAngle : Outport  Port=2  VectorParamsAs1DForOutWhenUnconnected=off
  RotorSpd : Outport  Port=3  VectorParamsAs1DForOutWhenUnconnected=off
  RotorAngle : Outport  Port=4  VectorParamsAs1DForOutWhenUnconnected=off
  RotorElecSpd : Outport  Port=5  VectorParamsAs1DForOutWhenUnconnected=off
  wires:
  [Tw_mode] -> Switch/2
  Calculate Speed/1(w) -> Switch/3
  w_input/1 -> Switch/1
  [f] -> Calculate Speed/5(f)
  [B] -> Calculate Speed/4(B)
  [J] -> Calculate Speed/3(J)
  [P] -> Product/2, Product1/2
  Demux1/10 -> [Tw_mode]  "Tw_mode"
  Machine Torque/1(MotorTrq) -> Calculate Speed/2(MotorTrq), MotorTrq/1
  Tload/1 -> Calculate Speed/1(Tload)
  Switch/1 -> Speed to Pos/1(Omega), RotorSpd/1, Product/1
  Demux1/9 -> [f]  "f"
  Demux1/8 -> [B]  "B"
  Demux1/7 -> [J]  "J"
  Demux1/5 -> Terminator3/1  "Llr"
  Demux1/4 -> Terminator2/1  "Rr"
  Demux1/3 -> Terminator1/1  "Lls"
  Demux1/2 -> Terminator/1  "Rs"
  Demux1/6 -> Machine Torque/6(Lm)  "Lm"
  Demux1/1 -> [P], Machine Torque/5(P)  "P"
  Config/1 -> Demux1/1
  Idq/1 -> Demux/1
  Demux/4 -> Machine Torque/4(Irq)
  Demux/3 -> Machine Torque/3(Ird)
  Demux/2 -> Machine Torque/2(Isq)
  Demux/1 -> Machine Torque/1(Isd)
  Speed to Pos/1(Theta) -> RotorMechAngle/1, Product1/1
  Product/1 -> RotorElecSpd/1
  Product1/1 -> RotorAngle/1

== system slrt_induction_2level_inverter/Induction Motor and 2-Level Inverter HDL Wrapper/Subsystem/Induction Motor HDL/IM HDL/IM Electromagnetic Discrete/Clarke Transform ==
  Abc : Inport
  Add : Sum  Inputs=++--  RndMeth=Simplest  OutDataTypeStr=Inherit: Same as first input
  Add1 : Sum  Inputs=+-  RndMeth=Simplest  OutDataTypeStr=Inherit: Same as first input
  Demux : Demux  Outputs=3
  Gain1 : Gain  Gain=sqrt(3)/3  RndMeth=Simplest  OutDataTypeStr=Inherit: Same as input  ParamDataTypeStr=Inherit: Same as input
  Gain5 : Gain  Gain=1/3  RndMeth=Simplest  OutDataTypeStr=Inherit: Same as input  ParamDataTypeStr=Inherit: Same as input
  Alpha : Outport  VectorParamsAs1DForOutWhenUnconnected=off
  Beta : Outport  Port=2  VectorParamsAs1DForOutWhenUnconnected=off
  wires:
  Gain1/1 -> Beta/1
  Gain5/1 -> Alpha/1
  Demux/3 -> Add/4, Add1/2
  Demux/2 -> Add/3, Add1/1
  Add1/1 -> Gain1/1
  Add/1 -> Gain5/1
  Demux/1 -> Add/1, Add/2
  Abc/1 -> Demux/1

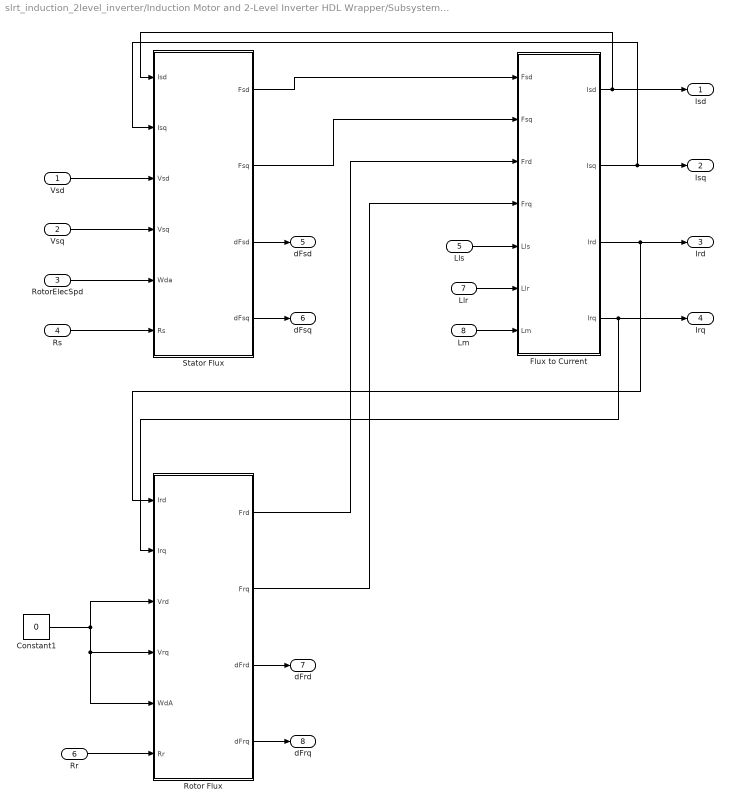
== system slrt_induction_2level_inverter/Induction Motor and 2-Level Inverter HDL Wrapper/Subsystem/Induction Motor HDL/IM HDL/IM Electromagnetic Discrete/IM Equivalent Circuit ==
  Vsd : Inport
  Vsq : Inport  Port=2
  RotorElecSpd : Inport  Port=3
  Rs : Inport  Port=4
  Lls : Inport  Port=5
  Rr : Inport  Port=6
  Llr : Inport  Port=7
  Lm : Inport  Port=8
  Constant1 : Constant  Value=0  OutDataTypeStr=Inherit: Inherit via back propagation  SampleTime=-1
  Flux to Current : Subsystem
  Rotor Flux : Subsystem
  Stator Flux : Subsystem
  Isd : Outport  VectorParamsAs1DForOutWhenUnconnected=off
  Isq : Outport  Port=2  VectorParamsAs1DForOutWhenUnconnected=off
  Ird : Outport  Port=3  VectorParamsAs1DForOutWhenUnconnected=off
  Irq : Outport  Port=4  VectorParamsAs1DForOutWhenUnconnected=off
  dFsd : Outport  Port=5  VectorParamsAs1DForOutWhenUnconnected=off
  dFsq : Outport  Port=6  VectorParamsAs1DForOutWhenUnconnected=off
  dFrd : Outport  Port=7  VectorParamsAs1DForOutWhenUnconnected=off
  dFrq : Outport  Port=8  VectorParamsAs1DForOutWhenUnconnected=off
  wires:
  Rr/1 -> Rotor Flux/6(Rr)
  Rs/1 -> Stator Flux/6(Rs)
  Lm/1 -> Flux to Current/7(Lm)
  Llr/1 -> Flux to Current/6(Llr)
  Lls/1 -> Flux to Current/5(Lls)
  Rotor Flux/4(dFrq) -> dFrq/1
  Rotor Flux/3(dFrd) -> dFrd/1
  Stator Flux/4(dFsq) -> dFsq/1
  Stator Flux/3(dFsd) -> dFsd/1
  Rotor Flux/2(Frq) -> Flux to Current/4(Frq)
  Rotor Flux/1(Frd) -> Flux to Current/3(Frd)
  Constant1/1 -> Rotor Flux/3(Vrd), Rotor Flux/4(Vrq), Rotor Flux/5(WdA)
  Vsd/1 -> Stator Flux/3(Vsd)
  Vsq/1 -> Stator Flux/4(Vsq)
  Stator Flux/2(Fsq) -> Flux to Current/2(Fsq)
  Stator Flux/1(Fsd) -> Flux to Current/1(Fsd)
  RotorElecSpd/1 -> Stator Flux/5(Wda)
  Flux to Current/4(Irq) -> Rotor Flux/2(Irq), Irq/1
  Flux to Current/3(Ird) -> Ird/1, Rotor Flux/1(Ird)
  Flux to Current/2(Isq) -> Isq/1, Stator Flux/2(Isq)
  Flux to Current/1(Isd) -> Isd/1, Stator Flux/1(Isd)

== system slrt_induction_2level_inverter/Induction Motor and 2-Level Inverter HDL Wrapper/Subsystem/Induction Motor HDL/IM HDL/IM Electromagnetic Discrete/Inverse Clarke Transform ==
  Alpha : Inport
  Beta : Inport  Port=2
  Gain1 : Gain  Gain=-sqrt(1/6)  RndMeth=Simplest  OutDataTypeStr=Inherit: Same as input  ParamDataTypeStr=Inherit: Same as input
  Gain2 : Gain  Gain=-sqrt(1/6)  RndMeth=Simplest  OutDataTypeStr=Inherit: Same as input  ParamDataTypeStr=Inherit: Same as input
  Gain3 : Gain  Gain=1/sqrt(2)  RndMeth=Simplest  OutDataTypeStr=Inherit: Same as input  ParamDataTypeStr=Inherit: Same as input
  Gain4 : Gain  Gain=-1/sqrt(2)  RndMeth=Simplest  OutDataTypeStr=Inherit: Same as input  ParamDataTypeStr=Inherit: Same as input
  Gain5 : Gain  Gain=sqrt(2/3)  RndMeth=Simplest  SaturateOnIntegerOverflow=on  OutDataTypeStr=Inherit: Same as input  ParamDataTypeStr=Inherit: Same as input
  Subtract1 : Sum  RndMeth=Simplest
  Subtract2 : Sum  RndMeth=Simplest
  A : Outport  VectorParamsAs1DForOutWhenUnconnected=off
  B : Outport  Port=2  VectorParamsAs1DForOutWhenUnconnected=off
  C : Outport  Port=3  VectorParamsAs1DForOutWhenUnconnected=off
  wires:
  Subtract2/1 -> C/1
  Subtract1/1 -> B/1
  Gain5/1 -> A/1
  Gain1/1 -> Subtract2/1
  Gain4/1 -> Subtract2/2
  Beta/1 -> Gain3/1, Gain4/1
  Alpha/1 -> Gain2/1, Gain1/1, Gain5/1
  Gain2/1 -> Subtract1/1
  Gain3/1 -> Subtract1/2

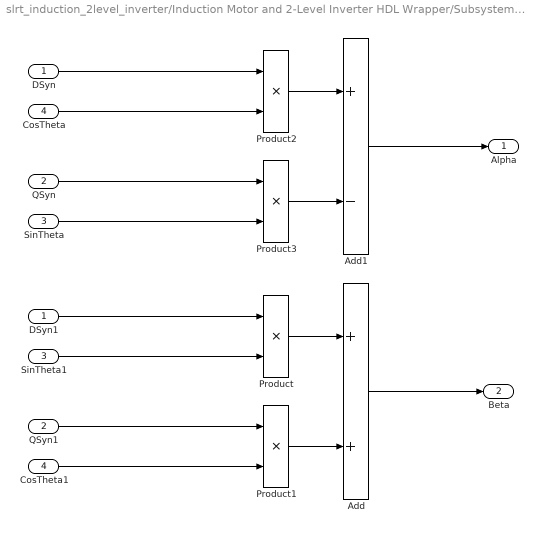
== system slrt_induction_2level_inverter/Induction Motor and 2-Level Inverter HDL Wrapper/Subsystem/Induction Motor HDL/IM HDL/IM Electromagnetic Discrete/Inverse Park Transform ==
  DSyn : Inport
  QSyn : Inport  Port=2
  SinTheta : Inport  Port=3
  CosTheta : Inport  Port=4
  Add : Sum  RndMeth=Simplest
  Add1 : Sum  Inputs=+-  RndMeth=Simplest
  CosTheta1 : InportShadow  Port=4
  DSyn1 : InportShadow
  Product{,1..3} (4 alike) : Product  RndMeth=Simplest
  QSyn1 : InportShadow  Port=2
  SinTheta1 : InportShadow  Port=3
  Alpha : Outport  VectorParamsAs1DForOutWhenUnconnected=off
  Beta : Outport  Port=2  VectorParamsAs1DForOutWhenUnconnected=off
  wires:
  Product/1 -> Add/1
  Product1/1 -> Add/2
  Add/1 -> Beta/1
  Product2/1 -> Add1/1
  Product3/1 -> Add1/2
  Add1/1 -> Alpha/1
  DSyn1/1 -> Product/1
  SinTheta1/1 -> Product/2
  CosTheta1/1 -> Product1/2
  QSyn1/1 -> Product1/1
  CosTheta/1 -> Product2/2
  QSyn/1 -> Product3/1
  SinTheta/1 -> Product3/2
  DSyn/1 -> Product2/1

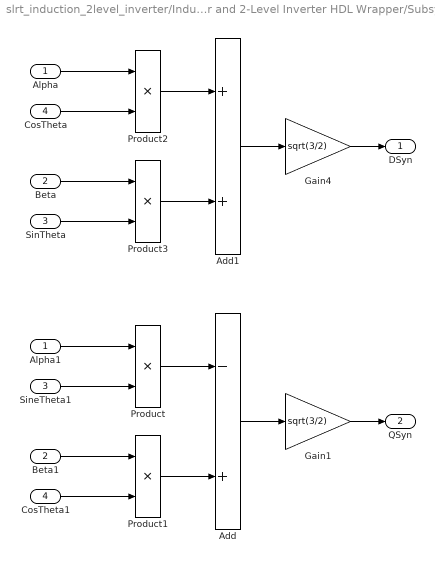
== system slrt_induction_2level_inverter/Induction Motor and 2-Level Inverter HDL Wrapper/Subsystem/Induction Motor HDL/IM HDL/IM Electromagnetic Discrete/Park Transform ==
  Alpha : Inport
  Beta : Inport  Port=2
  SinTheta : Inport  Port=3
  CosTheta : Inport  Port=4
  Add : Sum  Inputs=-+  OutDataTypeStr=Inherit: Same as first input
  Add1 : Sum  OutDataTypeStr=Inherit: Same as first input
  Alpha1 : InportShadow
  Beta1 : InportShadow  Port=2
  CosTheta1 : InportShadow  Port=4
  Gain1 : Gain  Gain=sqrt(3/2)  SaturateOnIntegerOverflow=on  OutDataTypeStr=Inherit: Same as input  ParamDataTypeStr=Inherit: Same as input
  Gain4 : Gain  Gain=sqrt(3/2)  SaturateOnIntegerOverflow=on  OutDataTypeStr=Inherit: Same as input  ParamDataTypeStr=Inherit: Same as input
  Product{,1..3} (4 alike) : Product  RndMeth=Zero  OutDataTypeStr=Inherit: Same as first input
  SineTheta1 : InportShadow  Port=3
  DSyn : Outport  VectorParamsAs1DForOutWhenUnconnected=off
  QSyn : Outport  Port=2  VectorParamsAs1DForOutWhenUnconnected=off
  wires:
  Gain1/1 -> QSyn/1
  Gain4/1 -> DSyn/1
  Product/1 -> Add/1
  Product1/1 -> Add/2
  Add/1 -> Gain1/1
  Product2/1 -> Add1/1
  Product3/1 -> Add1/2
  Add1/1 -> Gain4/1
  Alpha1/1 -> Product/1
  Beta1/1 -> Product1/1
  Alpha/1 -> Product2/1
  Beta/1 -> Product3/1
  CosTheta/1 -> Product2/2
  SinTheta/1 -> Product3/2
  SineTheta1/1 -> Product/2
  CosTheta1/1 -> Product1/2

== system slrt_induction_2level_inverter/Induction Motor and 2-Level Inverter HDL Wrapper/Subsystem/Induction Motor HDL/IM HDL/Mechanical and Angle/Calculate Speed ==
  Tload : Inport
  MotorTrq : Inport  Port=2
  J : Inport  Port=3
  B : Inport  Port=4
  f : Inport  Port=5
  Constant : Constant  Value=eps  OutDataTypeStr=Inherit: Inherit via back propagation  SampleTime=-1
  Data Type Duplicate : DataTypeDuplicate
  Discrete-Time Integrator : DiscreteIntegrator  SampleTime=-1  ICPrevOutput=DiscIntNeverNeededParam  ICPrevScaledInput=DiscIntNeverNeededParam
  Product : Product  Inputs=*/  RndMeth=Simplest  SaturateOnIntegerOverflow=on  OutDataTypeStr=Inherit: Same as first input
  Product1 : Product  Inputs=**  OutDataTypeStr=Inherit: Same as first input
  Product2 : Product  Inputs=**  OutDataTypeStr=Inherit: Same as first input
  Sign : Signum
  Sum1 : Sum  Inputs=-|+--
  Switch1 : Switch  Criteria=u2 ~= 0  SaturateOnIntegerOverflow=off  InputSameDT=off
  w : Outport
  wires:
  Constant/1 -> Data Type Duplicate/2, Switch1/3
  Switch1/1 -> Product/2
  J/1 -> Switch1/2, Switch1/1, Data Type Duplicate/1
  MotorTrq/1 -> Sum1/2
  Tload/1 -> Sum1/1
  f/1 -> Product2/2
  Product2/1 -> Sum1/4
  Sum1/1 -> Product/1
  Product/1 -> Discrete-Time Integrator/1
  Product1/1 -> Sum1/3
  Discrete-Time Integrator/1 -> Sign/1, Product1/1, w/1
  Sign/1 -> Product2/1
  B/1 -> Product1/2

== system slrt_induction_2level_inverter/Induction Motor and 2-Level Inverter HDL Wrapper/Subsystem/Induction Motor HDL/IM HDL/Mechanical and Angle/Machine Torque ==
  Isd : Inport
  Isq : Inport  Port=2
  Ird : Inport  Port=3
  Irq : Inport  Port=4
  P : Inport  Port=5
  Lm : Inport  Port=6
  Add : Sum  Inputs=+-  OutDataTypeStr=Inherit: Same as first input
  Product{,1,3..4} (4 alike) : Product  OutDataTypeStr=Inherit: Same as first input
  MotorTrq : Outport  VectorParamsAs1DForOutWhenUnconnected=off
  wires:
  Product4/1 -> Product3/2
  Product3/1 -> MotorTrq/1
  Lm/1 -> Product4/2
  P/1 -> Product4/1
  Add/1 -> Product3/1
  Irq/1 -> Product1/2
  Isd/1 -> Product1/1
  Ird/1 -> Product/2
  Isq/1 -> Product/1
  Product1/1 -> Add/2
  Product/1 -> Add/1

== system slrt_induction_2level_inverter/Induction Motor and 2-Level Inverter HDL Wrapper/Subsystem/Induction Motor HDL/IM HDL/Mechanical and Angle/Speed to Pos ==
  Omega : Inport
  Add : Sum  OutDataTypeStr=Inherit: Same as first input
  Add1 : Sum  OutDataTypeStr=Inherit: Same as first input
  Add2 : Sum  Inputs=+-  OutDataTypeStr=Inherit: Same as first input
  Compare To Constant : simulink/Logic and Bit Operations/Compare To Constant  relop=<=  const=U  OutDataTypeStr=boolean
  Compare To Constant1 : simulink/Logic and Bit Operations/Compare To Constant  relop=>=  const=L  OutDataTypeStr=boolean
  Constant : Constant  Value=U  OutDataTypeStr=Inherit: Inherit via back propagation  SampleTime=-1
  Constant2 : Constant  Value=L  OutDataTypeStr=Inherit: Inherit via back propagation  SampleTime=-1
  Data Type Duplicate : DataTypeDuplicate  NumInputPorts=4
  Data Type Duplicate1 : DataTypeDuplicate
  Delay : Delay  DelayLength=1
  Gain1 : Gain  Gain=Ts  OutDataTypeStr=Inherit: Same as input  ParamDataTypeStr=Inherit: Same as input
  Subtract : Sum  Inputs=+-  OutDataTypeStr=Inherit: Same as first input
  Switch : Switch  Criteria=u2 > Threshold  SaturateOnIntegerOverflow=off  InputSameDT=off
  Switch1 : Switch  Criteria=u2 > Threshold  SaturateOnIntegerOverflow=off  InputSameDT=off
  Theta : Outport  VectorParamsAs1DForOutWhenUnconnected=off
  wires:
  Omega/1 -> Gain1/1
  Compare To Constant/1 -> Switch/2
  Gain1/1 -> Add/1
  Compare To Constant1/1 -> Switch1/2
  Subtract/1 -> Switch/3
  Switch/1 -> Switch1/1
  Add1/1 -> Switch1/3
  Add2/1 -> Data Type Duplicate1/2, Subtract/2, Add1/2, Data Type Duplicate/1
  Add/1 -> Delay/1
  Delay/1 -> Switch/1, Data Type Duplicate1/1, Subtract/1, Compare To Constant1/1, Data Type Duplicate/2, Add1/1, Compare To Constant/1
  Switch1/1 -> Add/2, Theta/1
  Constant/1 -> Data Type Duplicate/3, Add2/1
  Constant2/1 -> Data Type Duplicate/4, Add2/2

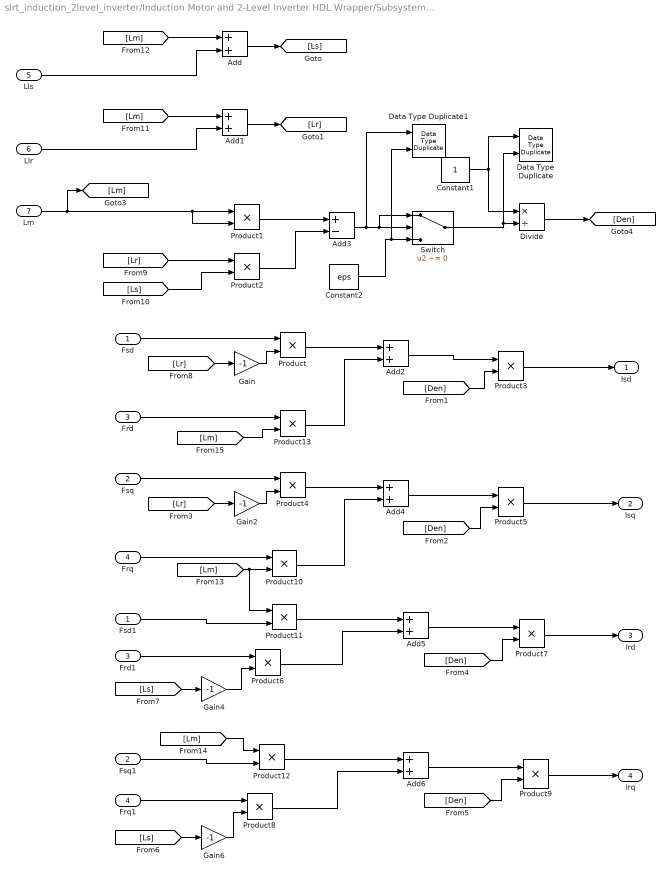
== system slrt_induction_2level_inverter/Induction Motor and 2-Level Inverter HDL Wrapper/Subsystem/Induction Motor HDL/IM HDL/IM Electromagnetic Discrete/IM Equivalent Circuit/Flux to Current ==
  Fsd : Inport
  Fsq : Inport  Port=2
  Frd : Inport  Port=3
  Frq : Inport  Port=4
  Lls : Inport  Port=5
  Llr : Inport  Port=6
  Lm : Inport  Port=7
  Add{,1..2,5..6} (5 alike) : Sum  RndMeth=Simplest  OutDataTypeStr=Inherit: Same as first input
  Add3 : Sum  Inputs=+-  RndMeth=Simplest  OutDataTypeStr=Inherit: Same as first input
  Add4 : Sum  OutDataTypeStr=Inherit: Same as first input
  Constant1 : Constant  VectorParams1D=off  OutDataTypeStr=Inherit: Inherit via back propagation  SampleTime=-1
  Constant2 : Constant  Value=eps  VectorParams1D=off  OutDataTypeStr=Inherit: Inherit via back propagation  SampleTime=-1
  Data Type Duplicate : DataTypeDuplicate
  Data Type Duplicate1 : DataTypeDuplicate
  Divide : Product  Inputs=*/  RndMeth=Simplest  SaturateOnIntegerOverflow=on  OutDataTypeStr=Inherit: Same as first input
  Frd1 : InportShadow  Port=3
  Frq1 : InportShadow  Port=4
  Fsd1 : InportShadow
  Fsq1 : InportShadow  Port=2
  Gain : Gain  Gain=-1  RndMeth=Simplest  OutDataTypeStr=Inherit: Same as input  ParamDataTypeStr=Inherit: Same as input
  Gain2 : Gain  Gain=-1  RndMeth=Simplest  OutDataTypeStr=Inherit: Same as input  ParamDataTypeStr=Inherit: Same as input
  Gain4 : Gain  Gain=-1  RndMeth=Simplest  OutDataTypeStr=Inherit: Same as input
  Gain6 : Gain  Gain=-1  RndMeth=Simplest  OutDataTypeStr=Inherit: Same as input
  Product{,1..2,4,6,8,10..13} (10 alike) : Product  RndMeth=Simplest  OutDataTypeStr=Inherit: Same as first input
  Product{3,5,7,9} (4 alike) : Product  RndMeth=Simplest  SaturateOnIntegerOverflow=on  OutDataTypeStr=Inherit: Same as first input
  Switch : Switch  Criteria=u2 ~= 0  SaturateOnIntegerOverflow=off  InputSameDT=off
  Isd : Outport  VectorParamsAs1DForOutWhenUnconnected=off
  Isq : Outport  Port=2  VectorParamsAs1DForOutWhenUnconnected=off
  Ird : Outport  Port=3  VectorParamsAs1DForOutWhenUnconnected=off
  Irq : Outport  Port=4  VectorParamsAs1DForOutWhenUnconnected=off
  wires:
  Constant2/1 -> Switch/3, Data Type Duplicate1/2
  Add3/1 -> Switch/2, Switch/1, Data Type Duplicate1/1
  Divide/1 -> [Den]
  [Lm] -> Product13/2
  Frd/1 -> Product13/1
  [Lm] -> Product12/1
  [Lm] -> Product10/2, Product11/1
  Frq/1 -> Product10/1
  [Den] -> Product3/2
  Constant1/1 -> Divide/1, Data Type Duplicate/1
  Switch/1 -> Divide/2, Data Type Duplicate/2
  Lls/1 -> Add/2
  Llr/1 -> Add1/2
  [Lm] -> Add/1
  Add/1 -> [Ls]
  [Lm] -> Add1/1
  Add1/1 -> [Lr]
  Fsd/1 -> Product/1
  [Lr] -> Gain/1
  Gain/1 -> Product/2
  Product/1 -> Add2/1
  Product13/1 -> Add2/2
  Lm/1 -> Product1/2, Product1/1, [Lm]
  [Lr] -> Product2/1
  [Ls] -> Product2/2
  Product1/1 -> Add3/1
  Product2/1 -> Add3/2
  Add2/1 -> Product3/1
  Product3/1 -> Isd/1
  Fsq/1 -> Product4/1
  [Lr] -> Gain2/1
  Gain2/1 -> Product4/2
  Product4/1 -> Add4/1
  Product10/1 -> Add4/2
  Add4/1 -> Product5/1
  [Den] -> Product5/2
  Product5/1 -> Isq/1
  [Ls] -> Gain4/1
  Gain4/1 -> Product6/2
  Add5/1 -> Product7/1
  [Den] -> Product7/2
  Product7/1 -> Ird/1
  [Ls] -> Gain6/1
  Gain6/1 -> Product8/2
  Add6/1 -> Product9/1
  [Den] -> Product9/2
  Product9/1 -> Irq/1
  Fsd1/1 -> Product11/2
  Product11/1 -> Add5/1
  Frd1/1 -> Product6/1
  Product6/1 -> Add5/2
  Fsq1/1 -> Product12/2
  Product12/1 -> Add6/1
  Frq1/1 -> Product8/1
  Product8/1 -> Add6/2

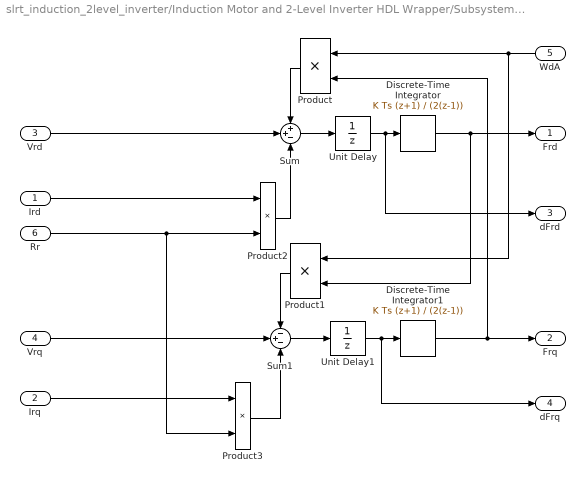
== system slrt_induction_2level_inverter/Induction Motor and 2-Level Inverter HDL Wrapper/Subsystem/Induction Motor HDL/IM HDL/IM Electromagnetic Discrete/IM Equivalent Circuit/Rotor Flux ==
  Ird : Inport
  Irq : Inport  Port=2
  Vrd : Inport  Port=3
  Vrq : Inport  Port=4
  WdA : Inport  Port=5
  Rr : Inport  Port=6
  Discrete-Time Integrator : DiscreteIntegrator  IntegratorMethod=Integration: Trapezoidal  SampleTime=Ts  RndMeth=Simplest  ICPrevOutput=DiscIntNeverNeededParam  ICPrevScaledInput=DiscIntNeverNeededParam
  Discrete-Time Integrator1 : DiscreteIntegrator  IntegratorMethod=Integration: Trapezoidal  SampleTime=Ts  RndMeth=Simplest  ICPrevOutput=DiscIntNeverNeededParam  ICPrevScaledInput=DiscIntNeverNeededParam
  Product : Product  InputSameDT=on  RndMeth=Zero  SaturateOnIntegerOverflow=on  OutDataTypeStr=Inherit: Same as first input
  Product1 : Product  InputSameDT=on  RndMeth=Zero  SaturateOnIntegerOverflow=on  OutDataTypeStr=Inherit: Same as first input
  Product2 : Product  RndMeth=Simplest  OutDataTypeStr=Inherit: Same as first input
  Product3 : Product  RndMeth=Simplest  OutDataTypeStr=Inherit: Same as first input
  Sum : Sum  Inputs=++-  InputSameDT=on  RndMeth=Simplest  SaturateOnIntegerOverflow=on  OutDataTypeStr=Inherit: Same as first input
  Sum1 : Sum  Inputs=-+-  InputSameDT=on  RndMeth=Simplest  SaturateOnIntegerOverflow=on  OutDataTypeStr=Inherit: Same as first input
  Unit Delay : UnitDelay  SampleTime=-1  HasFrameUpgradeWarning=on
  Unit Delay1 : UnitDelay  SampleTime=-1  HasFrameUpgradeWarning=on
  Frd : Outport  VectorParamsAs1DForOutWhenUnconnected=off
  Frq : Outport  Port=2  VectorParamsAs1DForOutWhenUnconnected=off
  dFrd : Outport  Port=3  VectorParamsAs1DForOutWhenUnconnected=off
  dFrq : Outport  Port=4  VectorParamsAs1DForOutWhenUnconnected=off
  wires:
  Unit Delay1/1 -> Discrete-Time Integrator1/1, dFrq/1
  Unit Delay/1 -> Discrete-Time Integrator/1, dFrd/1
  Rr/1 -> Product2/2, Product3/2
  Sum/1 -> Unit Delay/1
  Product/1 -> Sum/1
  WdA/1 -> Product/1, Product1/1
  Vrd/1 -> Sum/2
  Ird/1 -> Product2/1
  Product2/1 -> Sum/3
  Sum1/1 -> Unit Delay1/1
  Product1/1 -> Sum1/1
  Vrq/1 -> Sum1/2
  Irq/1 -> Product3/1
  Product3/1 -> Sum1/3
  Discrete-Time Integrator1/1 -> Product/2, Frq/1
  Discrete-Time Integrator/1 -> Frd/1, Product1/2
